simulink model "psd_model"  (R2013a)
settings: Solver=ode4  StartTime=0.0  StopTime=0.001  FixedStep=1e-9  RelTol=1e-3
libraries: powerlib x21
settings Model: Creator=ugurm  LastModifiedBy=mesutto

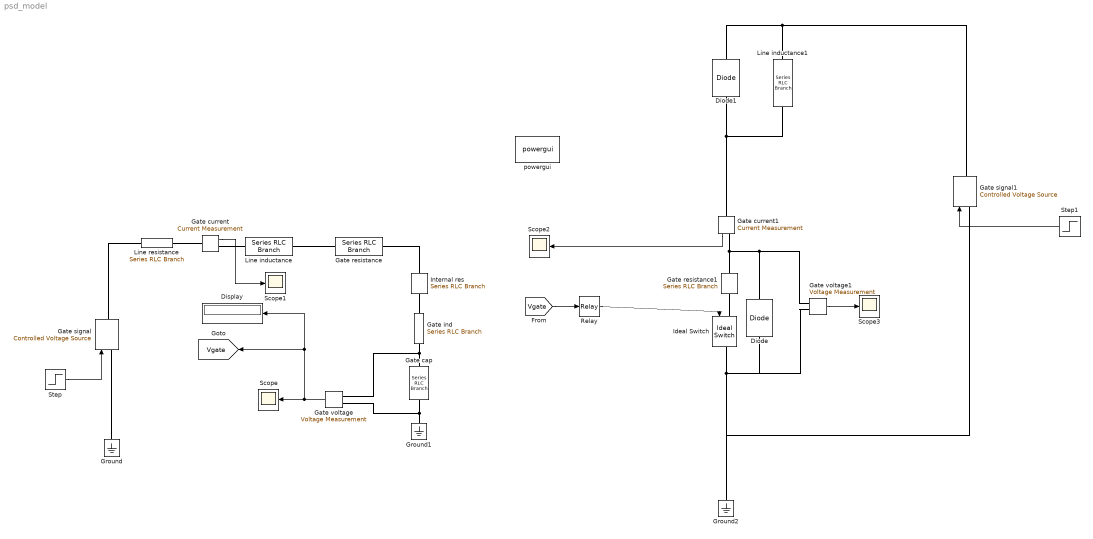
== system psd_model ==
  Diode : powerlib/Power Electronics/Diode  Ron=1e-9  Lon=0  Vf=1  IC=0  UseSnubber=off  Rs=1e15  Cs=1e-15  Measurements=off
  Diode1 : powerlib/Power Electronics/Diode  Ron=1e-9  Lon=0  Vf=1  IC=0  UseSnubber=off  Rs=1e15  Cs=1e-15  Measurements=off
  Display : Display
  Gate cap : powerlib/Elements/Series RLC Branch  LConnTagsString=__new0  RConnTagsString=__new0  BranchType=C  Resistance=4.7  Inductance=1e-3  SetiL0=off  InitialCurrent=0  Capacitance=1e-9  Setx0=off  InitialVoltage=0  Measurements=None
  Gate current : powerlib/Measurements/Current Measurement  PhasorSimulation=off  OutputType=Complex  PSBequivalent=0
  Gate current1 : powerlib/Measurements/Current Measurement  PhasorSimulation=off  OutputType=Complex  PSBequivalent=0
  Gate ind : powerlib/Elements/Series RLC Branch  LConnTagsString=__new0  RConnTagsString=__new0  BranchType=L  Resistance=10e-9  Inductance=10e-9  SetiL0=off  InitialCurrent=0  Capacitance=1e-6  Setx0=off  InitialVoltage=0  Measurements=None
  Gate resistance : powerlib/Elements/Series RLC Branch  LConnTagsString=__new0  RConnTagsString=__new0  BranchType=R  Resistance=4.7  Inductance=1e-3  SetiL0=off  InitialCurrent=0  Capacitance=1e-6  Setx0=off  InitialVoltage=0  Measurements=None
  Gate resistance1 : powerlib/Elements/Series RLC Branch  LConnTagsString=__new0  RConnTagsString=__new0  BranchType=R  Resistance=100e-3  Inductance=1e-3  SetiL0=off  InitialCurrent=0  Capacitance=1e-6  Setx0=off  InitialVoltage=0  Measurements=None
  Gate signal : powerlib/Electrical Sources/Controlled Voltage Source  Initialize=on  Source_Type=AC  Amplitude=0  Phase=0  Frequency=0  Measurements=None
  Gate signal1 : powerlib/Electrical Sources/Controlled Voltage Source  Initialize=on  Source_Type=AC  Amplitude=0  Phase=0  Frequency=0  Measurements=None
  Gate voltage : powerlib/Measurements/Voltage Measurement  PhasorSimulation=off  OutputType=Complex  PSBequivalent=0
  Gate voltage1 : powerlib/Measurements/Voltage Measurement  PhasorSimulation=off  OutputType=Complex  PSBequivalent=0
  Ground : powerlib/Elements/Ground  LConnTagsString=a
  Ground1 : powerlib/Elements/Ground  LConnTagsString=a
  Ground2 : powerlib/Elements/Ground  LConnTagsString=a
  Ideal Switch : powerlib/Power Electronics/Ideal Switch  Ron=1e-12  Lon=0  IC=0  Rs=1e15  Cs=inf  Measurements=off
  Internal res : powerlib/Elements/Series RLC Branch  LConnTagsString=__new0  RConnTagsString=__new0  BranchType=R  Resistance=1  Inductance=1e-3  SetiL0=off  InitialCurrent=0  Capacitance=1e-6  Setx0=off  InitialVoltage=0  Measurements=None
  Line inductance : powerlib/Elements/Series RLC Branch  LConnTagsString=__new0  RConnTagsString=__new0  BranchType=L  Resistance=10e-9  Inductance=100e-9  SetiL0=off  InitialCurrent=0  Capacitance=1e-6  Setx0=off  InitialVoltage=0  Measurements=None
  Line inductance1 : powerlib/Elements/Series RLC Branch  LConnTagsString=__new0  RConnTagsString=__new0  BranchType=L  Resistance=10e-9  Inductance=380e-6  SetiL0=off  InitialCurrent=0  Capacitance=1e-6  Setx0=off  InitialVoltage=0  Measurements=None
  Line resistance : powerlib/Elements/Series RLC Branch  LConnTagsString=__new0  RConnTagsString=__new0  BranchType=R  Resistance=1e-3  Inductance=1e-3  SetiL0=off  InitialCurrent=0  Capacitance=1e-6  Setx0=off  InitialVoltage=0  Measurements=None
  Relay : Relay  OnSwitchValue=2.5  OffSwitchValue=2.4
  Scope{,1..3} (4 alike) : Scope
      Scope settings: YMin=0  YMax=7.5  MaxDataPoints=22000
      Scope2 settings: YMin=0  YMax=7.5  SaveName=ScopeData2  MaxDataPoints=22000
      Scope3 settings: YMin=25  YMax=90  SaveName=ScopeData3  MaxDataPoints=22000
  Step : Step  Time=0.0001  After=5  SampleTime=0
  Step1 : Step  Time=0  After=400  SampleTime=0
  powergui : powerlib/powergui  Priority=1  SimulationMode=Discrete  SolverType=Tustin  SampleTime=1e-9  frequency=60  SPID=off  DisableSnubberDevices=off  DisableRonSwitches=off  DisableVfSwitches=off  SwTol=0  Interpol=off  DisplayEquations=off  frequencyindice=0  Pbase=100e6  ErrMax=1e-4  Iterations=50  UnitsV=kV  UnitsW=MW  FunctionMessages=off  echomessages=off  HookPort=off  EnableUseOfTLC=off  x0status=blocks  RestoreLinks=warning  ResistiveCurrentMeasurement=off  Frange=[0:2:500]  Ylog=off  Xlog=on  ShowGrid=off  save=off  variable=ZData  structure=idc  ZoomFFT=off  StartTime=0.1  cycles=20  DisplayStyle=5  fundamental=50  FreqAxis=off  MaxFrequency=20000  frequencyindicesteady=1  RmsSteady=1  display=off  Ts=0  methode=off
  tag scope: Vgate=global
  wires:
  Step/1 -> Gate signal/1
  Gate current/1 -> Scope1/1
  Gate voltage/1 -> Display/1, [Vgate], Scope/1
  Relay/1 -> Ideal Switch/1
  Step1/1 -> Gate signal1/1
  [Vgate] -> Relay/1
  Gate current1/1 -> Scope2/1
  Gate voltage1/1 -> Scope3/1
  connections:
  Line resistance/LConn1 -- Gate signal/RConn1
  Line inductance/RConn1 -- Gate resistance/LConn1
  Ground/LConn1 -- Gate signal/LConn1
  Gate ind/LConn1 -- Internal res/RConn1
  Ground1/LConn1 -- Gate cap/RConn1 -- Gate voltage/LConn2
  Gate cap/LConn1 -- Gate voltage/LConn1 -- Gate ind/RConn1
  Gate resistance/RConn1 -- Internal res/LConn1
  Gate current/LConn1 -- Line resistance/RConn1
  Gate current/RConn1 -- Line inductance/LConn1
  Ideal Switch/LConn1 -- Gate resistance1/RConn1
  Ideal Switch/RConn1 -- Diode/LConn1 -- Gate voltage1/LConn2 -- Ground2/LConn1 -- Gate signal1/LConn1
  Diode/RConn1 -- Gate voltage1/LConn1 -- Gate current1/RConn1 -- Gate resistance1/LConn1
  Gate current1/LConn1 -- Diode1/LConn1 -- Line inductance1/RConn1
  Diode1/RConn1 -- Line inductance1/LConn1 -- Gate signal1/RConn1
